simulink model "Eclipse_Unit_Test"  (R2018b)
settings: Solver=VariableStepAuto  StartTime=0.0  StopTime=5600  FixedStep=fswParams.sample_time_s  RelTol=1e-8  AbsTol=1e-8
undefined symbols (not defined in the file or in its folder): B_eci_unit, Conversion_lib, DiscIntNeverNeededParam, e2sun_eci_unit, ECLIPSE, env_acc_mps2, Environment_lib, fswParams, gyro_body_radps, gyro_meas_valid, mag_body_T, mag_meas_valid, MEKF_Conversion_lib, MEKF_lib, photodiodes_A, q_body, r_eci_km, satelliteDynamics_lib, sc2sun_eci_unit, Sensors_Lib, simParams, solar_panel_power_W, sun_sensor_lib, sunsensor_2body_lib, sunsensor_body_deg, sunsensor_body_rad, sunsensor_valid, v_eci_km, w_body_radps
libraries: aerolibutil x9, vrlib x6, simulink x5, sharedutil x4, magnetometer_lib x3, sharedtransform x2, dspmathops x2, gyroscope_lib x2, gravityGrad_Lib x1, atmoDrag_lib x1, magField_lib x1, solarPressure_lib x1
(part 2 of 2)

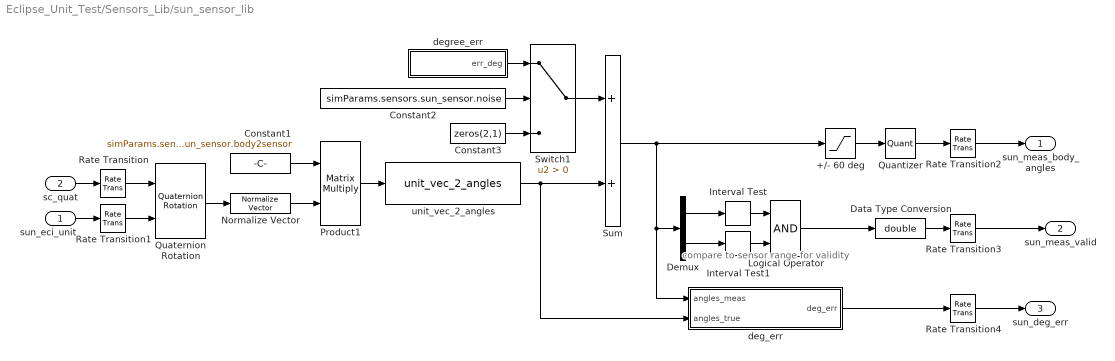
== system Eclipse_Unit_Test/Sensors_Lib/sun_sensor_lib  ==
  note: compare to sensor range for validity
  sun_eci_unit : Inport
  sc_quat : Inport  Port=2
  +/- 60 deg : Saturate  UpperLimit=simParams.sensors.sun_sensor.range_deg  LowerLimit=-simParams.sensors.sun_sensor.range_deg
  Constant1 : Constant  Value=simParams.sensors.sun_sensor.body2sensor
  Constant2 : Constant  Value=simParams.sensors.sun_sensor.noise
  Constant3 : Constant  Value=zeros(2,1)
  Data Type Conversion : DataTypeConversion  OutDataTypeStr=double
  Demux : Demux  Outputs=2
  Interval Test : simulink/Logic and Bit Operations/Interval Test  IntervalClosedRight=on  uplimit=simParams.sensors.sun_sensor.range_deg  IntervalClosedLeft=on  lowlimit=-simParams.sensors.sun_sensor.range_deg  OutDataTypeStr=boolean
  Interval Test1 : simulink/Logic and Bit Operations/Interval Test  IntervalClosedRight=on  uplimit=simParams.sensors.sun_sensor.range_deg  IntervalClosedLeft=on  lowlimit=-simParams.sensors.sun_sensor.range_deg  OutDataTypeStr=boolean
  Logical Operator : Logic  AllPortsSameDT=off  OutDataTypeStr=boolean
  Normalize Vector : vrlib/Utilities/Normalize Vector  maxzero=0
      settings: SourceProductName=Simulink 3D Animation  SourceProductBaseCode=VR
  Product1 : Product  Multiplication=Matrix(*)  RndMeth=Zero
  Quantizer : Quantizer  QuantizationInterval=simParams.sensors.sun_sensor.resolution
  Quaternion Rotation : aerolibutil/Quaternion Rotation
  Rate Transition : RateTransition  InitialCondition=simParams.initialConditions.q0  OutPortSampleTime=simParams.sensors.sun_sensor.sample_time_s
  Rate Transition1 : RateTransition  OutPortSampleTime=simParams.sensors.sun_sensor.sample_time_s
  Rate Transition2 : RateTransition
  Rate Transition3 : RateTransition
  Rate Transition4 : RateTransition
  Sum : Sum
  Switch1 : Switch  Criteria=u2 > Threshold
  deg_err : Subsystem
  degree_err : Subsystem
  unit_vec_2_angles : ss_vec_2_angles/unit_vec_2_angles  SystemSampleTime=-1
  sun_meas_body_angles : Outport
  sun_meas_valid : Outport  Port=2
  sun_deg_err : Outport  Port=3
  wires:
  Rate Transition4/1 -> sun_deg_err/1
  Rate Transition2/1 -> sun_meas_body_angles/1
  Rate Transition1/1 -> Quaternion Rotation/2
  Rate Transition/1 -> Quaternion Rotation/1
  Data Type Conversion/1 -> Rate Transition3/1
  Demux/2 -> Interval Test1/1
  Sum/1 -> Demux/1, deg_err/1(angles_meas), +/- 60 deg/1
  unit_vec_2_angles/1 -> deg_err/2(angles_true), Sum/2
  Product1/1 -> unit_vec_2_angles/1
  Constant1/1 -> Product1/1
  +/- 60 deg/1 -> Quantizer/1
  Logical Operator/1 -> Data Type Conversion/1
  Interval Test1/1 -> Logical Operator/2
  Interval Test/1 -> Logical Operator/1
  Demux/1 -> Interval Test/1
  Normalize Vector/1 -> Product1/2
  Quantizer/1 -> Rate Transition2/1
  Quaternion Rotation/1 -> Normalize Vector/1
  degree_err/1("err_deg ") -> Switch1/1
  deg_err/1(deg_err) -> Rate Transition4/1
  sun_eci_unit/1 -> Rate Transition1/1
  Switch1/1 -> Sum/1
  Constant3/1 -> Switch1/3
  Constant2/1 -> Switch1/2
  sc_quat/1 -> Rate Transition/1
  Rate Transition3/1 -> sun_meas_valid/1

== system Eclipse_Unit_Test/satelliteDynamics_lib/RigidBodyDynamics ==
  external_torque : Inport
  RW_torque : Inport  Port=2
  Integrator : Integrator  InitialCondition=[0;0;0]
  dynamics : Subsystem
  wint : Integrator  InitialCondition=[0.01;0.005;0]  AbsoluteTolerance=1e-10
  body_rates : Outport
  wires:
  external_torque/1 -> dynamics/1(external_torque_Nm)
  Integrator/1 -> dynamics/3(rw_momentum_Nms)
  RW_torque/1 -> Integrator/1, dynamics/2(rw_torque_Nm)
  dynamics/1(omega_dot) -> wint/1
  wint/1 -> dynamics/4(omega_radps), body_rates/1

== system Eclipse_Unit_Test/satelliteDynamics_lib/quat_propagation ==
  body_rates : Inport
  Gain1 : Gain  Gain=1/2
  Integrator : Integrator  InitialCondition=[0;0.707106781186547;0.707106781186547;0]
  MATLAB Function : MATLAB Function  TreatAsAtomicUnit=on
  Product : Product  Multiplication=Matrix(*)  RndMeth=Zero
  Quaternion Normalize : sharedutil/Quaternion Normalize  aMode=aMode
      settings: SourceProductName=Aerospace Blockset  SourceProductBaseCode=AE
  Scope : Scope
  quat : Outport
  wires:
  Quaternion Normalize/1 -> Scope/1, Product/2, quat/1
  Gain1/1 -> Product/1
  body_rates/1 -> MATLAB Function/1(w)
  MATLAB Function/1(Omega) -> Gain1/1
  Product/1 -> Integrator/1
  Integrator/1 -> Quaternion Normalize/1

== system Eclipse_Unit_Test/Conversion_lib/sunsensor_body_rad1/Create_Sz ==
  alpha : Inport
  beta : Inport  Port=2
  Constant : Constant
  Math Function : Math  Operator=square  SaturateOnIntegerOverflow=on
  Math Function1 : Math  Operator=square  SaturateOnIntegerOverflow=on
  Math Function2 : Math  Operator=reciprocal  SaturateOnIntegerOverflow=on
  Sqrt : Sqrt  SaturateOnIntegerOverflow=on
  Sum : Sum  Inputs=|+++
  Tan : Trigonometry  Operator=tan
  Tan1 : Trigonometry  Operator=tan
  Out1 : Outport
  wires:
  Constant/1 -> Sum/1
  Sum/1 -> Math Function2/1
  Tan/1 -> Math Function/1
  Math Function/1 -> Sum/2
  Math Function2/1 -> Sqrt/1
  Tan1/1 -> Math Function1/1
  alpha/1 -> Tan/1
  beta/1 -> Tan1/1
  Math Function1/1 -> Sum/3
  Sqrt/1 -> Out1/1

== system Eclipse_Unit_Test/MEKF_lib1/MEKF or Propagation/Angle_between_vectors ==
  sun_meas_rad_body : Inport
  mag_meas_T_body : Inport  Port=2
  Divide : Product  Inputs=*/
  Dot Product : DotProduct  InputSameDT=on  OutDataTypeStr=Inherit: Inherit via internal rule
  Dot Product1 : DotProduct  InputSameDT=on  OutDataTypeStr=Inherit: Inherit via internal rule
  Dot Product2 : DotProduct  InputSameDT=on  OutDataTypeStr=Inherit: Inherit via internal rule
  MATLAB Function : MATLAB Function  TreatAsAtomicUnit=on
  Multiply : Product
  Sqrt : Sqrt  SaturateOnIntegerOverflow=on
  Sqrt1 : Sqrt  SaturateOnIntegerOverflow=on
  Parallel_Protection : Outport
  wires:
  Dot Product1/1 -> Sqrt/1
  mag_meas_T_body/1 -> Dot Product2/2, Dot Product2/1, Dot Product/2
  sun_meas_rad_body/1 -> Dot Product1/1, Dot Product1/2, Dot Product/1
  Sqrt1/1 -> Multiply/2
  Sqrt/1 -> Multiply/1
  Dot Product/1 -> Divide/1
  Dot Product2/1 -> Sqrt1/1
  Multiply/1 -> Divide/2
  Divide/1 -> MATLAB Function/1(u)
  MATLAB Function/1(y) -> Parallel_Protection/1

== system Eclipse_Unit_Test/MEKF_lib1/Measurement Update/Subsystem ==
  sun_body_hat : Inport
  mag_body_hat : Inport  Port=2
  Constant1 : Constant  Value=zeros(3,3)  VectorParams1D=off
  Constant2 : Constant  Value=zeros(3,3)  VectorParams1D=off
  Cross_product_matrix2 : Subsystem
  Cross_product_matrix3 : Subsystem
  Horizontal Matrix Concatenate : Concatenate  Mode=Multidimensional array
  Horizontal Matrix Concatenate1 : Concatenate  Mode=Multidimensional array
  Vertical Matrix Concatenate : Concatenate  Mode=Multidimensional array  ConcatenateDimension=2
  H_matrix : Outport
  wires:
  Vertical Matrix Concatenate/1 -> H_matrix/1
  mag_body_hat/1 -> Cross_product_matrix3/1(mag_body_hat)
  Cross_product_matrix2/1(sun_body_x) -> Horizontal Matrix Concatenate/1
  sun_body_hat/1 -> Cross_product_matrix2/1(sun_body_hat)
  Horizontal Matrix Concatenate1/1 -> Vertical Matrix Concatenate/2
  Horizontal Matrix Concatenate/1 -> Vertical Matrix Concatenate/1
  Cross_product_matrix3/1(mag_body_x) -> Horizontal Matrix Concatenate/2
  Constant2/1 -> Horizontal Matrix Concatenate1/1
  Constant1/1 -> Horizontal Matrix Concatenate1/2

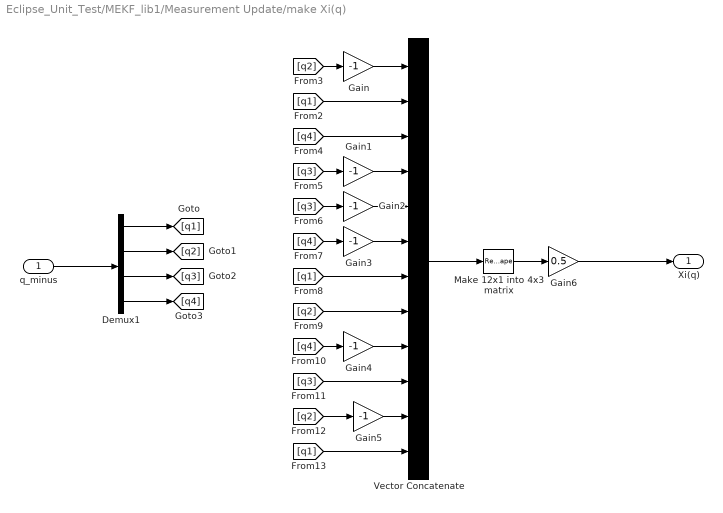
== system Eclipse_Unit_Test/MEKF_lib1/Measurement Update/make Xi(q) ==
  q_minus : Inport
  Demux1 : Demux
  Gain{,1..5} (6 alike) : Gain  Gain=-1
  Gain6 : Gain  Gain=0.5
  Make 12x1 into 4x3 matrix : Reshape  OutputDimensionality=Customize  OutputDimensions=[4,3]
  Vector Concatenate : Concatenate  NumInputs=12
  Xi(q) : Outport
  wires:
  Gain6/1 -> Xi(q)/1
  q_minus/1 -> Demux1/1
  Demux1/4 -> [q4]
  [q1] -> Vector Concatenate/7
  Gain5/1 -> Vector Concatenate/11
  [q4] -> Gain4/1
  [q2] -> Gain5/1
  Gain/1 -> Vector Concatenate/1
  [q1] -> Vector Concatenate/12
  [q4] -> Vector Concatenate/3
  Demux1/3 -> [q3]
  Gain4/1 -> Vector Concatenate/9
  Demux1/1 -> [q1]
  [q2] -> Vector Concatenate/8
  Demux1/2 -> [q2]
  Gain1/1 -> Vector Concatenate/4
  Gain2/1 -> Vector Concatenate/5
  [q3] -> Vector Concatenate/10
  [q2] -> Gain/1
  [q4] -> Gain3/1
  [q3] -> Gain1/1
  Make 12x1 into 4x3 matrix/1 -> Gain6/1
  [q1] -> Vector Concatenate/2
  Gain3/1 -> Vector Concatenate/6
  [q3] -> Gain2/1
  Vector Concatenate/1 -> Make 12x1 into 4x3 matrix/1

== system Eclipse_Unit_Test/MEKF_lib1/Subsystem/If Action Subsystem2 ==
  In1 : Inport
  Action Port : ActionPort
  Out1 : Outport
  wires:
  In1/1 -> Out1/1

== system Eclipse_Unit_Test/MEKF_lib1/Time Propagation (q,P)/Cross_Product_matrix ==
  omega_est : Inport
  Constant1 : Constant  Value=0
  Constant2 : Constant  Value=0
  Constant3 : Constant  Value=0
  Demux1 : Demux  Outputs=3
  Gain : Gain  Gain=-1
  Gain1 : Gain  Gain=-1
  Gain3 : Gain  Gain=-1
  Makes Cross Product Matrix : Reshape  OutputDimensionality=Customize  OutputDimensions=[3,3]
  Vector Concatenate : Concatenate  NumInputs=9
  omega_x : Outport
  wires:
  Vector Concatenate/1 -> Makes Cross Product Matrix/1
  Demux1/2 -> [v2]
  Demux1/1 -> [v1]
  Demux1/3 -> [v3]
  [v2] -> Vector Concatenate/7
  Constant3/1 -> Vector Concatenate/9
  [v1] -> Vector Concatenate/6
  omega_est/1 -> Demux1/1
  [v1] -> Gain1/1
  [v3] -> Vector Concatenate/2
  Constant1/1 -> Vector Concatenate/1
  Constant2/1 -> Vector Concatenate/5
  Makes Cross Product Matrix/1 -> omega_x/1
  [v3] -> Gain3/1
  [v2] -> Gain/1
  Gain/1 -> Vector Concatenate/3
  Gain3/1 -> Vector Concatenate/4
  Gain1/1 -> Vector Concatenate/8

== system Eclipse_Unit_Test/MEKF_lib1/Time Propagation (q,P)/Cross_product_matrix ==
  Psi_vec : Inport
  Constant1 : Constant  Value=0
  Constant2 : Constant  Value=0
  Constant3 : Constant  Value=0
  Demux1 : Demux  Outputs=3
  Gain : Gain  Gain=-1
  Gain1 : Gain  Gain=-1
  Gain3 : Gain  Gain=-1
  Makes Cross Product Matrix : Reshape  OutputDimensionality=Customize  OutputDimensions=[3,3]
  Vector Concatenate : Concatenate  NumInputs=9
  Psi_x : Outport
  wires:
  Constant3/1 -> Vector Concatenate/9
  [v3] -> Gain3/1
  [v2] -> Gain/1
  Demux1/3 -> [v3]
  Makes Cross Product Matrix/1 -> Psi_x/1
  Psi_vec/1 -> Demux1/1
  Gain/1 -> Vector Concatenate/3
  Gain1/1 -> Vector Concatenate/8
  Vector Concatenate/1 -> Makes Cross Product Matrix/1
  Demux1/2 -> [v2]
  [v3] -> Vector Concatenate/2
  Constant1/1 -> Vector Concatenate/1
  [v2] -> Vector Concatenate/7
  [v1] -> Vector Concatenate/6
  Constant2/1 -> Vector Concatenate/5
  Gain3/1 -> Vector Concatenate/4
  [v1] -> Gain1/1
  Demux1/1 -> [v1]

== system Eclipse_Unit_Test/MEKF_lib1/Time Propagation (q,P)/Psi ==
  del_t : Inport
  omega_vec : Inport  Port=2
  omega_mag : Inport  Port=3
  If : If  IfExpression=u1<1e-10
  If Action Subsystem : Subsystem  TreatAsAtomicUnit=on
  If Action Subsystem1 : Subsystem  TreatAsAtomicUnit=on
  Merge : Merge
  Psi1 : Outport
  wires:
  If/2 -> If Action Subsystem/Action
  If Action Subsystem/1(Psi) -> Merge/2
  If/1 -> If Action Subsystem1/Action
  If Action Subsystem1/1(Psi_zero) -> Merge/1
  Merge/1 -> Psi1/1
  omega_vec/1 -> If Action Subsystem/2(omega_vec)
  del_t/1 -> If Action Subsystem/1(del_t)
  omega_mag/1 -> If Action Subsystem/3(omega_mag), If/1

== system Eclipse_Unit_Test/MEKF_lib1/Time Propagation (q,P)/Subsystem ==
  del_t : Inport
  Psi_cross : Inport  Port=2
  Psi_vector : Inport  Port=3
  omega_magnitude : Inport  Port=4
  Add1 : Sum  Inputs=+-
  Constant : Constant  Value=0.5
  Cos : Trigonometry  Operator=cos
  Gain : Gain  Gain=-1
  Identity Matrix : S-Function  FunctionName=sdspeye  Parameters=Inherit,N,Ts,isCustomFloat,fxpIsSigned,dTypeID,fxpWordLength,fxpFracLength,1  SFunctionDeploymentMode=off  EnableBusSupport=off  mask(Identity Matrix){Inherit=off, N=3, Ts=1, additionalParams=off, allowOverrides=on, dataType=double, isSigned=on, wordLen=16, udDataType=sfix(16), fracBitsMode=Best precision, numFracBits=15, OutDataTypeStr=double, LastOutDataTypeStr=double}
      mask prompts: Inherit "Inherit output port attributes from input port"; N "Matrix size:"; Ts "Sample time:"; additionalParams "------- Show additional parameters --------"; allowOverrides "Allow overrides by DSP Fixed-Point Attributes blocks"; dataType "Output data type:"; isSigned "Signed"; wordLen "Word length:"; udDataType "User-defined data type (e.g. sfix(16), float('single')):"; fracBitsMode "Set fraction length in output to:"; numFracBits "Fraction length:"; OutDataTypeStr "Output data type:"; LastOutDataTypeStr "Last output data type:"
      mask help: Output an identity matrix. If the matrix size entered is a scalar, then the output will be a square (symmetric) identity matrix with the number of rows and columns both equal to the specified value. If the matrix size entered is a two-element vector [M N], then the output will be an asymmetric matrix with the number of rows equal to M, the number of columns equal to N, ones down the diagonal, and zeros elsewhere. This matches the syntax of the MATLAB function eye(N) and eye(M,N), respectively.
      mask init:
      | isCustomFloat =  0; % nice default
      | fxpIsSigned   =  1; % nice default
      | fxpWordLength =  8; % nice default
      | fxpFracLength =  0; % nice default
      | if Inherit
      |     dTypeID   = -3; % SAME_AS_INPUT
      | else
      |     dtRows            = dspblkGetDiscreteImpulseDTRowInfo();
      |     [dtInfo, dTypeID] = dspblkUDTMapperOutDType(gcbh, dtRows{1}, 'dataType', 1.0);
      |     isCustomFloat     = dtInfo.DataTypeIsCustomFloat;
      |     if ~isCustomFloat
      |         fxpIsSigned   = dtInfo.DataTypeIsSigned;
      |         fxpWordLength = dtInfo.DataTypeWordLength;
      |         fxpFracLength = dtInfo.DataTypeFracOrMantBits;
      |     end
      | end
      mask Help: eval('blocksethelp');
      mask Callback Inherit: dspblkeye
      mask TypeOptions dataType: double | single | int8 | uint8 | int16 | uint16 | int32 | uint32 | boolean | Fixed-point | User-defined | Inherit via back propagation
      mask TypeOptions fracBitsMode: Best precision | User-defined
      mask Display:
      | if Inherit
      |     disp('eye( )');
      | else
      |     disp(['eye(' , num2str(get_param(gcbh, 'N')), ')']);
      | end
  Matrix Concatenate : Concatenate  Mode=Multidimensional array  ConcatenateDimension=2
  Matrix Concatenate1 : Concatenate  Mode=Multidimensional array  ConcatenateDimension=2
  Matrix Concatenate2 : Concatenate  Mode=Multidimensional array
  Matrix Multiply2 : Product
  Multiply : Product  Inputs=3
  Transpose2 : Math  Operator=transpose  SaturateOnIntegerOverflow=on
  OMEGA : Outport
  wires:
  Matrix Concatenate2/1 -> OMEGA/1
  Multiply/1 -> Cos/1
  Matrix Multiply2/1 -> Add1/1
  Add1/1 -> Matrix Concatenate1/2
  Matrix Concatenate1/1 -> Matrix Concatenate2/2
  Matrix Concatenate/1 -> Matrix Concatenate2/1
  Psi_vector/1 -> Gain/1, Matrix Concatenate1/1
  Cos/1 -> Matrix Concatenate/1, Matrix Multiply2/1
  Transpose2/1 -> Matrix Concatenate/2
  Psi_cross/1 -> Add1/2
  Identity Matrix/1 -> Matrix Multiply2/2
  del_t/1 -> Multiply/1
  omega_magnitude/1 -> Multiply/3
  Constant/1 -> Multiply/2
  Gain/1 -> Transpose2/1

== system Eclipse_Unit_Test/MEKF_lib1/Triad/Angle_between_vectors ==
  sun_meas_rad_body : Inport
  mag_meas_T_body : Inport  Port=2
  Divide : Product  Inputs=*/
  Dot Product : DotProduct  InputSameDT=on  OutDataTypeStr=Inherit: Inherit via internal rule
  Dot Product1 : DotProduct  InputSameDT=on  OutDataTypeStr=Inherit: Inherit via internal rule
  Dot Product2 : DotProduct  InputSameDT=on  OutDataTypeStr=Inherit: Inherit via internal rule
  MATLAB Function : MATLAB Function  TreatAsAtomicUnit=on
  Multiply : Product
  Sqrt : Sqrt  SaturateOnIntegerOverflow=on
  Sqrt1 : Sqrt  SaturateOnIntegerOverflow=on
  Parallel_Protection : Outport
  wires:
  Dot Product1/1 -> Sqrt/1
  mag_meas_T_body/1 -> Dot Product2/2, Dot Product2/1, Dot Product/2
  sun_meas_rad_body/1 -> Dot Product1/1, Dot Product1/2, Dot Product/1
  Sqrt1/1 -> Multiply/2
  Sqrt/1 -> Multiply/1
  Dot Product/1 -> Divide/1
  Dot Product2/1 -> Sqrt1/1
  Multiply/1 -> Divide/2
  Divide/1 -> MATLAB Function/1(u)
  MATLAB Function/1(y) -> Parallel_Protection/1

== system Eclipse_Unit_Test/MEKF_lib1/Triad/Bypass Triad ==
  quat_old : Inport
  Action Port : ActionPort
  quat_new : Outport
  wires:
  quat_old/1 -> quat_new/1

== system Eclipse_Unit_Test/MEKF_lib1/Triad/Triad_alg ==
  sun_body : Inport
  mag_body : Inport  Port=2
  "mag_inertial " : Inport  Port=3
  sun_inertial : Inport  Port=4
  Action Port : ActionPort
  Cross Product{4..7} (4 alike) : vrlib/Utilities/Cross Product
      settings: SourceProductBaseCode=VR
  Direction Cosine Matrix to Quaternions2 : sharedtransform/Direction Cosine Matrix  to Quaternions  aMode=0  action=None  tolerance=eps(2)
      settings: SourceProductName=Aerospace Blockset  SourceProductBaseCode=AE
  Math Function1 : Math  Operator=transpose  SaturateOnIntegerOverflow=on
  Matrix Concatenate2 : Concatenate  NumInputs=3  Mode=Multidimensional array  ConcatenateDimension=2
  Matrix Concatenate3 : Concatenate  NumInputs=3  Mode=Multidimensional array  ConcatenateDimension=2
  Matrix Multiply1 : Product  Multiplication=Matrix(*)
  Multiply : Product
  Normalization6 : dspmathops/Normalization  NormType=2-norm  Bias=1e-10  NormOver=Each column  Dimension=1  roundingMode=Floor  overflowMode=off  accumDataTypeStr=Inherit: Same as product output  accumLastDataTypeStr=Inherit: Same as product output  outputDataTypeStr=Inherit: Same as product output  outputMin=[]  outputMax=[]  outputLastDataTypeStr=Inherit: Same as product output
      settings: SourceProductName=DSP System Toolbox
  Normalization7 : dspmathops/Normalization  NormType=2-norm  Bias=1e-10  NormOver=Each column  Dimension=1  roundingMode=Floor  overflowMode=off  accumDataTypeStr=Inherit: Same as product output  accumLastDataTypeStr=Inherit: Same as product output  outputDataTypeStr=Inherit: Same as product output  outputMin=[]  outputMax=[]  outputLastDataTypeStr=Inherit: Same as product output
      settings: SourceProductName=DSP System Toolbox
  Selector : Selector  InputPortWidth=4  IndexOptions=Index vector (dialog)  Indices=[1]  OutputSizes=1
  Sign : Signum
  quat_out 2 : Outport
  wires:
  sun_body/1 -> Matrix Concatenate2/1, Cross Product5/1, Cross Product4/1
  mag_body/1 -> Cross Product4/2
  Cross Product4/1 -> Normalization6/1  "S x M"
  Normalization6/1 -> Matrix Concatenate2/2, Cross Product5/2  "M"
  Cross Product5/1 -> Matrix Concatenate2/3  "S x M"
  sun_inertial/1 -> Cross Product6/1, Matrix Concatenate3/1, Cross Product7/1
  Cross Product7/1 -> Matrix Concatenate3/3  "S x M"
  Normalization7/1 -> Matrix Concatenate3/2, Cross Product7/2  "M"
  Cross Product6/1 -> Normalization7/1  "S x M"
  "mag_inertial "/1 -> Cross Product6/2
  Matrix Concatenate3/1 -> Math Function1/1
  Matrix Multiply1/1 -> Direction Cosine Matrix to Quaternions2/1
  Matrix Concatenate2/1 -> [dcm_body]
  Math Function1/1 -> [dcm_Inert]
  [dcm_body] -> Matrix Multiply1/1
  [dcm_Inert] -> Matrix Multiply1/2
  Direction Cosine Matrix to Quaternions2/1 -> Multiply/2, Selector/1
  Sign/1 -> Multiply/1
  Selector/1 -> Sign/1
  Multiply/1 -> quat_out 2/1

== system Eclipse_Unit_Test/Sensors_Lib/gyroscope_array/gyroscope_lib ==
  note: check the value of omega against
      | the programmed measurement range
      | of the sensor
  omega_in_radps : Inport
  ARW : Gain  Gain=simParams.sensors.gyro.arw(id_s)
  Cast To Double : DataTypeConversion  OutDataTypeStr=double
  Check Static Range : simulink/Model Verification/Check  Static Range  Description=simParams.sensors.gyro.w_min(id_s) <= u <= simParams.sensors.gyro.w_max(id_s)  max=simParams.sensors.gyro.w_max(id_s)  max_included=on  min=simParams.sensors.gyro.w_min(id_s)  min_included=on  enabled=on  stopWhenAssertionFail=off  export=on  icon=graphic
      settings: SourceProductName=Simulink  SourceProductBaseCode=SL
  Check Static Range1 : simulink/Model Verification/Check  Static Range  Description=simParams.sensors.gyro.w_min(id_s) <= u <= simParams.sensors.gyro.w_max(id_s)  max=simParams.sensors.gyro.w_max(id_s)  max_included=on  min=simParams.sensors.gyro.w_min(id_s)  min_included=on  enabled=on  stopWhenAssertionFail=off  export=on  icon=graphic
      settings: SourceProductName=Simulink  SourceProductBaseCode=SL
  Check Static Range2 : simulink/Model Verification/Check  Static Range  Description=simParams.sensors.gyro.w_min(id_s) <= u <= simParams.sensors.gyro.w_max(id_s)  max=simParams.sensors.gyro.w_max(id_s)  max_included=on  min=simParams.sensors.gyro.w_min(id_s)  min_included=on  enabled=on  stopWhenAssertionFail=off  export=on  icon=graphic
      settings: SourceProductName=Simulink  SourceProductBaseCode=SL
  Demux : Demux  Outputs=3
  Discrete-Time Integrator : DiscreteIntegrator  InitialCondition=simParams.sensors.gyro.bias_init(id_s)  SampleTime=-1  ICPrevOutput=DiscIntNeverNeededParam  ICPrevScaledInput=DiscIntNeverNeededParam
  Logical Operator : Logic  Inputs=3  AllPortsSameDT=off  OutDataTypeStr=boolean
  Quantizer1 : Quantizer  QuantizationInterval=simParams.sensors.gyro.resolution(id_s)
  Quantizer2 : Quantizer  QuantizationInterval=simParams.sensors.gyro.resolution(id_s)
  RRW : Gain  Gain=simParams.sensors.gyro.rrw(id_s)
  Random Number : RandomNumber  Mean=[0 0 0]  Variance=[1 1 1]  Seed=simParams.sensors.gyro.seed_arw(:,id_s)  SampleTime=simParams.sensors.gyro.sample_time_s
  Random Number1 : RandomNumber  Mean=[0 0 0]  Variance=[1 1 1]  Seed=simParams.sensors.gyro.seed_rrw(:,id_s)  SampleTime=simParams.sensors.gyro.sample_time_s
  Rate Transition : RateTransition  InitialCondition=simParams.initialConditions.w0  OutPortSampleTime=simParams.sensors.gyro.sample_time_s
  Rate Transition1 : RateTransition  InitialCondition=simParams.initialConditions.w0
  Rate Transition2 : RateTransition  InitialCondition=simParams.sensors.gyro.bias_init(id_s)
  Rate Transition3 : RateTransition  InitialCondition=1
  Scope : Scope
  Sum : Sum  Inputs=|++
  Sum1 : Sum  Inputs=|++
  omega_radps : Outport
  bias_out : Outport  Port=2
  gyro_valid : Outport  Port=3
  wires:
  Logical Operator/1 -> Cast To Double/1
  Check Static Range2/1 -> Logical Operator/3
  Check Static Range/1 -> Logical Operator/1
  Check Static Range1/1 -> Logical Operator/2
  Demux/1 -> Check Static Range/1
  Demux/2 -> Check Static Range1/1
  Demux/3 -> Check Static Range2/1
  Rate Transition3/1 -> gyro_valid/1
  Rate Transition2/1 -> bias_out/1
  Rate Transition1/1 -> Scope/1, omega_radps/1
  Rate Transition/1 -> Sum/1, Demux/1
  Quantizer2/1 -> Rate Transition1/1
  Sum1/1 -> Quantizer2/1
  Quantizer1/1 -> Sum/2
  Discrete-Time Integrator/1 -> Sum1/2, Rate Transition2/1
  Cast To Double/1 -> Rate Transition3/1
  RRW/1 -> Discrete-Time Integrator/1
  Sum/1 -> Sum1/1
  omega_in_radps/1 -> Rate Transition/1
  ARW/1 -> Quantizer1/1
  Random Number1/1 -> RRW/1
  Random Number/1 -> ARW/1

== system Eclipse_Unit_Test/Sensors_Lib/sun_sensor_lib /deg_err ==
  note: Computes the norm of the 2x1 degree error vector
  angles_meas : Inport
  angles_true : Inport  Port=2
  Dot Product : DotProduct  InputSameDT=on  OutDataTypeStr=Inherit: Inherit via internal rule
  Sqrt : Sqrt  SaturateOnIntegerOverflow=on
  Sum : Sum  Inputs=+-
  deg_err : Outport
  wires:
  Sqrt/1 -> deg_err/1
  Dot Product/1 -> Sqrt/1
  Sum/1 -> Dot Product/1, Dot Product/2
  angles_true/1 -> Sum/2
  angles_meas/1 -> Sum/1

== system Eclipse_Unit_Test/Sensors_Lib/sun_sensor_lib /degree_err ==
  Mux : Mux  Inputs=2
  Random Number2 : RandomNumber  Variance=simParams.sensors.sun_sensor.deg_var  Seed=simParams.sensors.sun_sensor.seed(1)  SampleTime=simParams.sensors.sun_sensor.sample_time_s
  Random Number3 : RandomNumber  Variance=simParams.sensors.sun_sensor.deg_var  Seed=simParams.sensors.sun_sensor.seed(2)  SampleTime=simParams.sensors.sun_sensor.sample_time_s
  "err_deg " : Outport
  wires:
  Mux/1 -> "err_deg "/1
  Random Number3/1 -> Mux/2
  Random Number2/1 -> Mux/1

== system Eclipse_Unit_Test/satelliteDynamics_lib/RigidBodyDynamics/dynamics ==
  note: Euler's equation: J dw/dt = T_{ext} + T_{rw} - w x ( Jw + h_w )
      |
      | RW being momentum exchange devices do NOT create
      | an external torque on the s/c
  external_torque_Nm : Inport
  rw_torque_Nm : Inport  Port=2
  rw_momentum_Nms : Inport  Port=3
  omega_radps : Inport  Port=4
  Add : Sum  Inputs=|++
  Cross Product : vrlib/Utilities/Cross Product
      settings: SourceProductBaseCode=VR
  Invert  3x3 Matrix : aerolibutil/Invert  3x3 Matrix
  Product : Product  Multiplication=Matrix(*)  RndMeth=Zero
  Product1 : Product  Multiplication=Matrix(*)  RndMeth=Zero
  Sum : Sum  Inputs=+-+
  inertia_tensor1 : Constant  Value=simParams.scParams.J
  inertia_tensor2 : Constant  Value=simParams.scParams.J
  omega_dot : Outport
  wires:
  rw_momentum_Nms/1 -> Add/2
  external_torque_Nm/1 -> Sum/1
  omega_radps/1 -> Product/2, Cross Product/1
  inertia_tensor2/1 -> Product/1
  Sum/1 -> Product1/2
  Product1/1 -> omega_dot/1
  Invert  3x3 Matrix/1 -> Product1/1
  inertia_tensor1/1 -> Invert  3x3 Matrix/1
  Cross Product/1 -> Sum/2
  Product/1 -> Add/1
  Add/1 -> Cross Product/2
  rw_torque_Nm/1 -> Sum/3

== system Eclipse_Unit_Test/MEKF_lib1/Measurement Update/Subsystem/Cross_product_matrix2 ==
  sun_body_hat : Inport
  Constant1 : Constant  Value=0
  Constant2 : Constant  Value=0
  Constant3 : Constant  Value=0
  Demux1 : Demux  Outputs=3
  Gain1 : Gain  Gain=-1
  Gain3 : Gain  Gain=-1
  Gain4 : Gain  Gain=-1
  Makes Cross Product Matrix : Reshape  OutputDimensionality=Customize  OutputDimensions=[3,3]
  Vector Concatenate : Concatenate  NumInputs=9
  sun_body_x : Outport
  wires:
  Gain1/1 -> Vector Concatenate/8
  Gain4/1 -> Vector Concatenate/4
  [v2] -> Gain3/1
  Constant1/1 -> Vector Concatenate/1
  [v1] -> Gain1/1
  Gain3/1 -> Vector Concatenate/3
  sun_body_hat/1 -> Demux1/1
  [v3] -> Vector Concatenate/2
  [v2] -> Vector Concatenate/7
  Demux1/2 -> [v2]
  Constant2/1 -> Vector Concatenate/5
  Vector Concatenate/1 -> Makes Cross Product Matrix/1
  Demux1/3 -> [v3]
  [v3] -> Gain4/1
  Constant3/1 -> Vector Concatenate/9
  [v1] -> Vector Concatenate/6
  Demux1/1 -> [v1]
  Makes Cross Product Matrix/1 -> sun_body_x/1

== system Eclipse_Unit_Test/MEKF_lib1/Measurement Update/Subsystem/Cross_product_matrix3 ==
  mag_body_hat : Inport
  Constant1 : Constant  Value=0
  Constant2 : Constant  Value=0
  Constant3 : Constant  Value=0
  Demux1 : Demux  Outputs=3
  Gain1 : Gain  Gain=-1
  Gain3 : Gain  Gain=-1
  Gain4 : Gain  Gain=-1
  Makes Cross Product Matrix : Reshape  OutputDimensionality=Customize  OutputDimensions=[3,3]
  Vector Concatenate : Concatenate  NumInputs=9
  mag_body_x : Outport
  wires:
  mag_body_hat/1 -> Demux1/1
  [v1] -> Vector Concatenate/6
  [v2] -> Vector Concatenate/7
  Gain3/1 -> Vector Concatenate/3
  [v3] -> Gain4/1
  [v3] -> Vector Concatenate/2
  Demux1/1 -> [v1]
  Gain1/1 -> Vector Concatenate/8
  Constant1/1 -> Vector Concatenate/1
  [v1] -> Gain1/1
  Makes Cross Product Matrix/1 -> mag_body_x/1
  Demux1/3 -> [v3]
  Constant2/1 -> Vector Concatenate/5
  Vector Concatenate/1 -> Makes Cross Product Matrix/1
  Demux1/2 -> [v2]
  Gain4/1 -> Vector Concatenate/4
  Constant3/1 -> Vector Concatenate/9
  [v2] -> Gain3/1

== system Eclipse_Unit_Test/MEKF_lib1/Time Propagation (q,P)/Psi/If Action Subsystem ==
  del_t : Inport
  omega_vec : Inport  Port=2
  omega_mag : Inport  Port=3
  Action Port : ActionPort
  Constant : Constant  Value=0.5
  Divide : Product  Inputs=***
  Divide1 : Product  Inputs=**/
  Sin : Trigonometry
  Psi : Outport
  wires:
  Divide1/1 -> Psi/1  "Psi"
  omega_mag/1 -> Divide1/3, Divide/3
  Constant/1 -> Divide/2
  omega_vec/1 -> Divide1/2
  Divide/1 -> Sin/1
  del_t/1 -> Divide/1
  Sin/1 -> Divide1/1  "sin(om_mag*0.5*del_t)"

== system Eclipse_Unit_Test/MEKF_lib1/Time Propagation (q,P)/Psi/If Action Subsystem1 ==
  Action Port : ActionPort
  Constant : Constant  Value=0
  Constant1 : Constant  Value=0
  Constant2 : Constant  Value=0
  Mux : Mux  Inputs=3
  Psi_zero : Outport
  wires:
  Constant/1 -> Mux/1
  Constant1/1 -> Mux/2
  Constant2/1 -> Mux/3
  Mux/1 -> Psi_zero/1

== matlab function Eclipse_Unit_Test/satelliteDynamics_lib/quat_propagation/MATLAB Function ==
  data: w input; Omega output
function Omega = skew_sym(w)
%#codegen

    w_skew = ...
        [0 w(3) -w(2);
        -w(3) 0 w(1);
        w(2) -w(1) 0];

    Omega = ...
        [0 -w';
        w w_skew];

== matlab function Eclipse_Unit_Test/MEKF_lib1/MEKF or Propagation/Angle_between_vectors/MATLAB Function ==
  data: u input; y output
function y = fcn(u)
%#codegen
if abs(u) <=  cosd(2.5)
    y = 1;
else
y = 0;
end

== matlab function Eclipse_Unit_Test/MEKF_lib1/Triad/Angle_between_vectors/MATLAB Function ==
  data: u input; y output
function y = fcn(u)
%#codegen
if abs(u) <=  cosd(2.5)
    y = 1;
else
y = 0;
end

== matlab function Eclipse_Unit_Test/MEKF_lib1/Measurement Update/QR Factorization ==
  data: P_sq output; R_sq input; K output; P_sq input; gyro_valid input; H input
function [P_sq,K] = A_QR(R_sq,P_sq, gyro_valid,H)
%#codegen
[nr,~] = size(R_sq);
[np,~] = size(P_sq);
A_QR = [R_sq',zeros(nr,np);(P_sq')*H', P_sq'];

[~,R] = qr(A_QR);
        P_sq = R(7:12,7:12)'; %Updated P_sq
        K_bar = R(1:6,7:12)';    
        Innovation_sq = R(1:6,1:6)';
        
        K = K_bar/(Innovation_sq);
        
        if( gyro_valid == 0 )
    K(4:6,:) = zeros(3,6); %this is done so that we do not update bias based
                            % on false gyro readings
        end
end

== matlab function Eclipse_Unit_Test/MEKF_lib1/Time Propagation (q,P)/MATLAB Function10 ==
  data: om_mag input; omega_x input; dt input; Phi output
function Phi = Phi_disc(om_mag,omega_x,dt)
%#codegen
% State Transition Matrix
w_n     = om_mag;
w_skew  = omega_x;

if( w_n < 1e-10 )
    Phi = [ eye(3)     -eye(3)*dt;
            zeros(3,3)  eye(3) ];
else
    Phi_11  = eye(3) - w_skew*(sin(w_n*dt)/w_n) + ...
                                        w_skew^2*(1 - cos(w_n*dt))/w_n^2;
    Phi_12  = w_skew*(1 - cos(w_n*dt))/w_n^2 - eye(3)*dt - ...
                                    w_skew^2*(w_n*dt - sin(w_n*dt))/w_n^3;
    Phi_21  = zeros(3,3);    
    Phi_22  = eye(3);    
    Phi     = [ Phi_11 Phi_12;
                Phi_21 Phi_22 ];
end

== matlab function Eclipse_Unit_Test/MEKF_lib1/Time Propagation (q,P)/MATLAB Function ==
  data: P_sq input; Phi_discrete input; P_sq output; Q_sq input
function P_sq  = Cqr(P_sq,Phi_discrete,Q_sq)
%#codegen

A_QR2 = [P_sq'*Phi_discrete';Q_sq'];
         [~,R2] = qr(A_QR2);
          sq_P_kp1 = R2(1:6,1:6)';
          P_sq = sq_P_kp1;
end
